simulink model "sldemo_tableplot_org"  (Simulink 10.0)
settings: Solver=ode2  StartTime=0.0  StopTime=22  FixedStep=.008  RelTol=1e-3
PreLoadFcn:
  | load sldemo_tableplot_data;
  | tabfig = figure;
  | hda = daexplr;
  | set(hda, 'position', [6 458 1077 544] );
  | set( tabfig, 'Position', [550, 415, 674, 510] );
InitFcn:
  | mh = get_param('sldemo_tableplot','object');
  | luth = get_param('sldemo_tableplot/2-D Lookup Table','object');
  | hda.view(mh);
  | hda.view(luth);
StopFcn:
  | sldemo_tableplot_comet(luth,logsOut);
undefined symbols (not defined in the file): one, two
Description:
  | Interpolation Algorithm Selection and Trajectory Animation
  | 
  | This example shows how to use a dynamic comet plot to visualize the result
  | of changing the interpolation and extrapolation options for a 2-D data set running
  | in an-D Lookup Table block.  Algorithm options can be employed in different
  | situations to tradeoff accuracy, smoothness, data size, and performance.
  | 
  | Try opening the model and using the lookup table block's dialog to
  | change the interpolation and extrapolation algorithms. A copy of the
  | dialog is embedded in the right hand pane in the  Model Explorer and
  | will show up after the first simulation.  You can enter and tweak values for
  | the entire model and its blocks from the Model Explorer, including settings
  | for model configuration parameters, Simulink blocks, Stateflow(R) charts, and
  | Simulink(R) Coder(TM) settings for code generation and data management.
  | 
  | To make the plot, data from the simulation is logged using the non-intrusive
  | logging features.  Non-intrusive logging is annotated on the block diagram
  | by the small blue "transmitter antennas" on certain block output ports.
  | These logging points can be set in three ways: from the MATLAB(R) command line
  | using set_param(), from the Diagram > Signals & Ports > Signal & Scope Manager, and
  | from the signal properties dialog.
CloseFcn:
  | if exist('hda')
  |   hide(hda);
  |   clear('hda');
  | end
  | if exist('tabfig')
  |   if ishghandle(tabfig, 'figure')
  |       close(tabfig);
  |   end
  |   clear('tabfig');
  | end
  | clear('luth');
settings Model: FPTRunName=Active  Creator=The MathWorks, Inc.  LastModifiedBy=bhisma  ExtModeTrigMode=oneshot  ExtModeArmWhenConnect=off  ExtModeAutoUpdateStatusClock=off
settings DataIOCC: SaveOutput=off  SaveTime=off  SignalLoggingName=logsOut
settings OptimizationCC: BlockReduction=off  BooleanDataType=off  ExpressionDepthLimit=2147483647  InitFltsAndDblsToZero=on
settings DebuggingCC: SaveWithParameterizedLinksMsg=none  UnderspecifiedInitializationDetection=Simplified  MergeDetectMultiDrivingBlocksExec=error  CheckExecutionContextPreStartOutputMsg=on  CheckExecutionContextRuntimeOutputMsg=on  SignalResolutionControl=TryResolveAllWithWarning  MultiTaskDSMMsg=warning  MultiTaskCondExecSysMsg=none  SigSpecEnsureSampleTimeMsg=none  FcnCallInpInsideContextMsg=warning  StateNameClashWarn=warning
settings HardwareCC: TargetUnknown=on
settings GRTTargetCC: TargetFcnLib=ansi_tfl_tmw.mat  GeneratePreprocessorConditionals=Disable all
settings ConfigComp: CovExternalEMLEnable=off  CovSFcnEnable=off

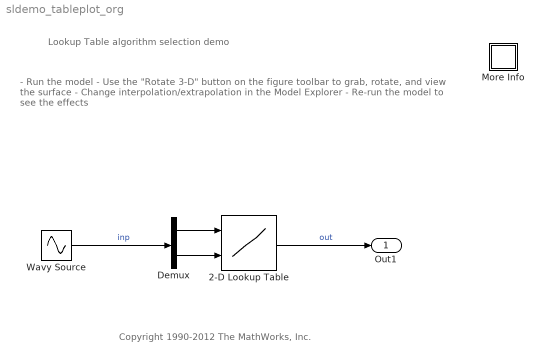
== system sldemo_tableplot_org ==
  note: - Run the model
      | - Use the "Rotate 3-D" button on the figure toolbar
      |   to grab, rotate, and view the surface
      | - Change interpolation/extrapolation in the Model Explorer
      | - Re-run the model to see the effects
  note: Lookup Table algorithm selection demo
  note: Copyright 1990-2012 The MathWorks, Inc.
  2-D Lookup Table : Lookup_n-D  BreakpointsForDimension1=one  BreakpointsForDimension2=two  Table=tab'  RndMeth=Simplest  InputSameDT=on
      settings: AttributesFormatString=interpolation: %<interpMethod>\nextrapolation: %<extrapMethod>
  Demux : Demux  Outputs=2
  More Info : Subsystem
      settings: OpenFcn=showdemo(bdroot(gcb))
      mask Display: disp('?')
  Wavy Source : Sin  Amplitude=[22.5, 25]  Bias=[22.5, 45]  Frequency=[1.714, 1]  Phase=[pi, 0]  SampleTime=0
  Out1 : Outport  VectorParamsAs1DForOutWhenUnconnected=off
  wires:
  2-D Lookup Table/1 -> Out1/1  "out"
  Wavy Source/1 -> Demux/1  "inp"
  Demux/1 -> 2-D Lookup Table/1
  Demux/2 -> 2-D Lookup Table/2

== system sldemo_tableplot_org/More Info ==
